simulink model "ALL_JP360_DBW_V6_5_1103"  (R2022a)
settings: Solver=FixedStepAuto  StartTime=0.0  StopTime=inf  FixedStep=0.01  RelTol=1e-3  EnableMultiTasking=on
model workspace (MAT data in the model file):
  g = 9.8
undefined symbols (not defined in the file or in its folder): canChannel, delta_v_p, IPM_Line_C0, IPM_Line_C1, IPM_Line_C2, IPM_Line_C3, M, M_p, MRR_ObjDistX, MRR_ObjDistY, MRR_ObjFusionCamID, MRR_ObjFusionSig, MRR_ObjID, MRR_ObjRelVelX, MRR_ObjRelVelY, MRR_ObjType, MRR_ObjUpdFlg, none, obj_vaild, untracktime, V, videoinput
libraries: canfdmsglib x230, canfdlib x76, slpidlib x24, simulink x18, dspstat3 x14, ctrlSharedLib x1, simulink_extras x1, imaqlib x1, realtime_pacer_lib x1, dspvision x1, visionsinks x1
(part 39 of 55)

== system ALL_JP360_DBW_V6_5_1103/MsgFromCAN/SRR_ADCU_MsgFromCAN/SRR_ADCU_RRR_OBJPos9_0x1BC ==
  SRR_ADCU_RRR_OBJPos9_0x1BCFromInData : Inport  OutDataTypeStr=Bus:CAN_FD_MESSAGE_BUS
  Bus Creator : BusCreator  Inputs=42  OutDataTypeStr=Bus:SRR_ADCU_RRR_OBJPos9_0x1BC  NonVirtualBus=on
  CAN FD Unpack : canfdmsglib/CAN FD Unpack  CANdbFile=V363 SRR Private CAN-V1.3.dbc  MsgList=(none)  MsgName=RRR_OBJPos9_0x1BC  ProtocolMode=CAN FD  MsgIDType=Standard (11-bit identifier)  MsgIdentifier=444  MsgLength=48  SignalInfo={'RRR_CRCCheck_0x1BC','376','16','BE','unsigned','Standard','0','1','0','0','65535';'RRR_OBJ17_Dx','79','13','BE','unsigned','Standard','0','0.0625','-256','-256','255.938';'RRR_OBJ17_Dy','60','11','BE','unsigned','Standard','0','0.125','-128','-128','127.875';'RRR_OBJ17_ExistProb','112','6','BE','unsigned','Standard','0','2','0','0','100';'RRR_OBJ17_HeadingAngle','55','10','BE','unsigned','Standard','0','0.01','-3.14','-3.14','3.14';'RRR_OBJ17_Height','26','9','BE','unsigned','Standard','0','0.01','0','0','5.11';'RRR_OBJ17_Length','33','9','BE','unsigned','Standard','0','0.05','0','0','25.5';'RRR_OBJ17_Measured','126','2','BE','unsigned','Standard','0','1','0','0','3';'RRR_OBJ17_Motion_Status','162','3','BE','unsigned','Standard','0','1','0','0','7';'RRR_OBJ17_ObstacleProb','120','6','BE','unsigned','Standard','0','2','0','0','100';'RRR_OBJ17_RefPointDx','144','13','BE','unsigned','Standard','0','0.0625','-256','-256','255.938';'RRR_OBJ17_RefPointDy','141','11','BE','unsigned','Standard','0','0.125','-128','-128','127.875';'RRR_OBJ17_RefPointLoc','157','3','BE','unsigned','Standard','0','1','0','0','7';'RRR_OBJ17_RelAx','118','9','BE','unsigned','Standard','0','0.0625','-16','-16','15.9375';'RRR_OBJ17_RelAy','111','10','BE','unsigned','Standard','0','0.03125','-16','-16','15.9688';'RRR_OBJ17_RelVx','89','12','BE','unsigned','Standard','0','0.0625','-128','-128','127.938';'RRR_OBJ17_RelVy','85','10','BE','unsigned','Standard','0','0.125','-64','-64','63.875';'RRR_OBJ17_Track_Age','165','8','BE','unsigned','Standard','0','1','0','0','255';'RRR_OBJ17_Track_ID','1','7','BE','unsigned','Standard','0','1','0','0','127';'RRR_OBJ17_Type','14','3','BE','unsigned','Standard','0','1','0','0','7';'RRR_OBJ17_Width','19','11','BE','unsigned','Standard','0','0.01','0','0','12';'RRR_OBJ18_Dx','247','13','BE','unsigned','Standard','0','0.0625','-256','-256','255.938';'RRR_OBJ18_Dy','228','11','BE','unsigned','Standard','0','0.125','-128','-128','127.875';'RRR_OBJ18_ExistProb','280','6','BE','unsigned','Standard','0','2','0','0','100';'RRR_OBJ18_HeadingAngle','223','10','BE','unsigned','Standard','0','0.01','-3.14','-3.14','3.14';'RRR_OBJ18_Height','194','9','BE','unsigned','Standard','0','0.01','0','0','5.11';'RRR_OBJ18_Length','201','9','BE','unsigned','Standard','0','0.05','0','0','25.5';'RRR_OBJ18_Measured','294','2','BE','unsigned','Standard','0','1','0','0','3';'RRR_OBJ18_Motion_Status','330','3','BE','unsigned','Standard','0','1','0','0','7';'RRR_OBJ18_ObstacleProb','288','6','BE','unsigned','Standard','0','2','0','0','100';'RRR_OBJ18_RefPointDx','312','13','BE','unsigned','Standard','0','0.0625','-256','-256','255.938';'RRR_OBJ18_RefPointDy','309','11','BE','unsigned','Standard','0','0.125','-128','-128','127.875';'RRR_OBJ18_RefPointLoc','325','3','BE','unsigned','Standard','0','1','0','0','7';'RRR_OBJ18_RelAx','286','9','BE','unsigned','Standard','0','0.0625','-16','-16','15.9375';'RRR_OBJ18_RelAy','279','10','BE','unsigned','Standard','0','0.03125','-16','-16','15.9688';'RRR_OBJ18_RelVx','257','12','BE','unsigned','Standard','0','0.0625','-128','-128','127.938';'RRR_OBJ18_RelVy','253','10','BE','unsigned','Standard','0','0.125','-64','-64','63.875';'RRR_OBJ18_Track_Age','333','8','BE','unsigned','Standard','0','1','0','0','255';'RRR_OBJ18_Track_ID','169','7','BE','unsigned','Standard','0','1','0','0','127';'RRR_OBJ18_Type','182','3','BE','unsigned','Standard','0','1','0','0','7';'RRR_OBJ18_Width','187','11','BE','unsigned','Standard','0','0.01','0','0','12';'RRR_RollingCounter_0x1BC','360','4','BE','unsigned','Standard','0','1','0','0','15'}  IDPort=off  TimestampPort=off  ErrorPort=off  RemotePort=off  LengthPort=off  StatusPort=off  BRSPort=off  ESIPort=off  DLCPort=off  ApplyMinMax=off
      settings: SourceProductBaseCode=ME,XP,VN  DataFormat=CANdb specified signals
  Data Type Conversion1 : DataTypeConversion  OutDataTypeStr=uint16  SaturateOnIntegerOverflow=off  RndMeth=Floor
  Data Type Conversion{4,8..10,13,19..20,24,28..30,33,39..40,42} (15 alike) : DataTypeConversion  OutDataTypeStr=int8  SaturateOnIntegerOverflow=off  RndMeth=Floor
  Data Type Conversion{2..3,5..7,11..12,14..17,21..23,25..27,31..32,34..37,41} (24 alike) : DataTypeConversion  OutDataTypeStr=single  SaturateOnIntegerOverflow=off  RndMeth=Floor
  Data Type Conversion18 : DataTypeConversion  OutDataTypeStr=uint8  SaturateOnIntegerOverflow=off  RndMeth=Floor
  Data Type Conversion38 : DataTypeConversion  OutDataTypeStr=uint8  SaturateOnIntegerOverflow=off  RndMeth=Floor
  SRR_ADCU_RRR_OBJPos9_0x1BCFromOutData : Outport  OutDataTypeStr=Bus:SRR_ADCU_RRR_OBJPos9_0x1BC
  wires:
  CAN FD Unpack/1 -> Data Type Conversion1/1
  CAN FD Unpack/2 -> Data Type Conversion2/1
  CAN FD Unpack/3 -> Data Type Conversion3/1
  CAN FD Unpack/4 -> Data Type Conversion4/1
  CAN FD Unpack/5 -> Data Type Conversion5/1
  CAN FD Unpack/6 -> Data Type Conversion6/1
  CAN FD Unpack/7 -> Data Type Conversion7/1
  CAN FD Unpack/8 -> Data Type Conversion8/1
  CAN FD Unpack/9 -> Data Type Conversion9/1
  CAN FD Unpack/10 -> Data Type Conversion10/1
  CAN FD Unpack/11 -> Data Type Conversion11/1
  CAN FD Unpack/12 -> Data Type Conversion12/1
  CAN FD Unpack/13 -> Data Type Conversion13/1
  CAN FD Unpack/14 -> Data Type Conversion14/1
  CAN FD Unpack/15 -> Data Type Conversion15/1
  CAN FD Unpack/16 -> Data Type Conversion16/1
  CAN FD Unpack/17 -> Data Type Conversion17/1
  CAN FD Unpack/18 -> Data Type Conversion18/1
  CAN FD Unpack/19 -> Data Type Conversion19/1
  CAN FD Unpack/20 -> Data Type Conversion20/1
  CAN FD Unpack/21 -> Data Type Conversion21/1
  CAN FD Unpack/22 -> Data Type Conversion22/1
  CAN FD Unpack/23 -> Data Type Conversion23/1
  CAN FD Unpack/24 -> Data Type Conversion24/1
  CAN FD Unpack/25 -> Data Type Conversion25/1
  CAN FD Unpack/26 -> Data Type Conversion26/1
  CAN FD Unpack/27 -> Data Type Conversion27/1
  CAN FD Unpack/28 -> Data Type Conversion28/1
  CAN FD Unpack/29 -> Data Type Conversion29/1
  CAN FD Unpack/30 -> Data Type Conversion30/1
  CAN FD Unpack/31 -> Data Type Conversion31/1
  CAN FD Unpack/32 -> Data Type Conversion32/1
  CAN FD Unpack/33 -> Data Type Conversion33/1
  CAN FD Unpack/34 -> Data Type Conversion34/1
  CAN FD Unpack/35 -> Data Type Conversion35/1
  CAN FD Unpack/36 -> Data Type Conversion36/1
  CAN FD Unpack/37 -> Data Type Conversion37/1
  CAN FD Unpack/38 -> Data Type Conversion38/1
  CAN FD Unpack/39 -> Data Type Conversion39/1
  CAN FD Unpack/40 -> Data Type Conversion40/1
  CAN FD Unpack/41 -> Data Type Conversion41/1
  CAN FD Unpack/42 -> Data Type Conversion42/1
  Data Type Conversion1/1 -> Bus Creator/1  "RRR_CRCCheck_0x1BC"
  Data Type Conversion2/1 -> Bus Creator/2  "RRR_OBJ17_Dx"
  Data Type Conversion3/1 -> Bus Creator/3  "RRR_OBJ17_Dy"
  Data Type Conversion4/1 -> Bus Creator/4  "RRR_OBJ17_ExistProb"
  Data Type Conversion5/1 -> Bus Creator/5  "RRR_OBJ17_HeadingAngle"
  Data Type Conversion6/1 -> Bus Creator/6  "RRR_OBJ17_Height"
  Data Type Conversion7/1 -> Bus Creator/7  "RRR_OBJ17_Length"
  Data Type Conversion8/1 -> Bus Creator/8  "RRR_OBJ17_Measured"
  Data Type Conversion9/1 -> Bus Creator/9  "RRR_OBJ17_Motion_Status"
  Data Type Conversion10/1 -> Bus Creator/10  "RRR_OBJ17_ObstacleProb"
  Data Type Conversion11/1 -> Bus Creator/11  "RRR_OBJ17_RefPointDx"
  Data Type Conversion12/1 -> Bus Creator/12  "RRR_OBJ17_RefPointDy"
  Data Type Conversion13/1 -> Bus Creator/13  "RRR_OBJ17_RefPointLoc"
  Data Type Conversion14/1 -> Bus Creator/14  "RRR_OBJ17_RelAx"
  Data Type Conversion15/1 -> Bus Creator/15  "RRR_OBJ17_RelAy"
  Data Type Conversion16/1 -> Bus Creator/16  "RRR_OBJ17_RelVx"
  Data Type Conversion17/1 -> Bus Creator/17  "RRR_OBJ17_RelVy"
  Data Type Conversion18/1 -> Bus Creator/18  "RRR_OBJ17_Track_Age"
  Data Type Conversion19/1 -> Bus Creator/19  "RRR_OBJ17_Track_ID"
  Data Type Conversion20/1 -> Bus Creator/20  "RRR_OBJ17_Type"
  Data Type Conversion21/1 -> Bus Creator/21  "RRR_OBJ17_Width"
  Data Type Conversion22/1 -> Bus Creator/22  "RRR_OBJ18_Dx"
  Data Type Conversion23/1 -> Bus Creator/23  "RRR_OBJ18_Dy"
  Data Type Conversion24/1 -> Bus Creator/24  "RRR_OBJ18_ExistProb"
  Data Type Conversion25/1 -> Bus Creator/25  "RRR_OBJ18_HeadingAngle"
  Data Type Conversion26/1 -> Bus Creator/26  "RRR_OBJ18_Height"
  Data Type Conversion27/1 -> Bus Creator/27  "RRR_OBJ18_Length"
  Data Type Conversion28/1 -> Bus Creator/28  "RRR_OBJ18_Measured"
  Data Type Conversion29/1 -> Bus Creator/29  "RRR_OBJ18_Motion_Status"
  Data Type Conversion30/1 -> Bus Creator/30  "RRR_OBJ18_ObstacleProb"
  Data Type Conversion31/1 -> Bus Creator/31  "RRR_OBJ18_RefPointDx"
  Data Type Conversion32/1 -> Bus Creator/32  "RRR_OBJ18_RefPointDy"
  Data Type Conversion33/1 -> Bus Creator/33  "RRR_OBJ18_RefPointLoc"
  Data Type Conversion34/1 -> Bus Creator/34  "RRR_OBJ18_RelAx"
  Data Type Conversion35/1 -> Bus Creator/35  "RRR_OBJ18_RelAy"
  Data Type Conversion36/1 -> Bus Creator/36  "RRR_OBJ18_RelVx"
  Data Type Conversion37/1 -> Bus Creator/37  "RRR_OBJ18_RelVy"
  Data Type Conversion38/1 -> Bus Creator/38  "RRR_OBJ18_Track_Age"
  Data Type Conversion39/1 -> Bus Creator/39  "RRR_OBJ18_Track_ID"
  Data Type Conversion40/1 -> Bus Creator/40  "RRR_OBJ18_Type"
  Data Type Conversion41/1 -> Bus Creator/41  "RRR_OBJ18_Width"
  Data Type Conversion42/1 -> Bus Creator/42  "RRR_RollingCounter_0x1BC"
  Bus Creator/1 -> SRR_ADCU_RRR_OBJPos9_0x1BCFromOutData/1  "SRR_ADCU_RRR_OBJPos9_0x1BCFromOutData"
  SRR_ADCU_RRR_OBJPos9_0x1BCFromInData/1 -> CAN FD Unpack/1  "SRR_ADCU_RRR_OBJPos9_0x1BCFromInData"

== system ALL_JP360_DBW_V6_5_1103/MsgFromCAN/Subsystem/Subsystem1 ==
  VR_ADCU_MRR_ObjHeader_0x680FromOutData : Inport
  Bus Selector : BusSelector  OutputSignals=MRR_ObjDistX_03,MRR_ObjDistY_03,MRR_ObjExistProb_03,MRR_ObjFusionCamID_03,MRR_ObjFusionSig_03,MRR_ObjID_03,MRR_ObjMovingSts_03,MRR_ObjObstacleProb_03,MRR_ObjRelAccelX_03,MRR_ObjRelAccelY_03,MRR_ObjRelVelX_03,MRR_ObjRelVelY_03,MRR_ObjType_03,MRR_ObjUpdFlg_03
  Bus Selector1 : BusSelector  OutputSignals=MRR_ObjDistX_04,MRR_ObjDistY_04,MRR_ObjExistProb_04,MRR_ObjFusionCamID_04,MRR_ObjFusionSig_04,MRR_ObjID_04,MRR_ObjMovingSts_04,MRR_ObjObstacleProb_04,MRR_ObjRelAccelX_04,MRR_ObjRelAccelY_04,MRR_ObjRelVelX_04,MRR_ObjRelVelY_04,MRR_ObjType_04,MRR_ObjUpdFlg_04
  Data Type Conversion{,1..27} (28 alike) : DataTypeConversion  OutDataTypeStr=single  SaturateOnIntegerOverflow=off  RndMeth=Floor
  Mux : Mux  Inputs=14
  Mux1 : Mux  Inputs=14
  Out1 : Outport
  Out2 : Outport  Port=2
  wires:
  Data Type Conversion26/1 -> Mux1/13
  Data Type Conversion24/1 -> Mux1/11
  Data Type Conversion22/1 -> Mux1/9
  Data Type Conversion20/1 -> Mux1/7
  Data Type Conversion27/1 -> Mux1/14
  Data Type Conversion25/1 -> Mux1/12
  Data Type Conversion23/1 -> Mux1/10
  Data Type Conversion21/1 -> Mux1/8
  Data Type Conversion13/1 -> Mux/14
  Data Type Conversion15/1 -> Mux1/2
  Data Type Conversion17/1 -> Mux1/4
  Data Type Conversion19/1 -> Mux1/6
  Data Type Conversion2/1 -> Mux/3
  Data Type Conversion14/1 -> Mux1/1
  Data Type Conversion16/1 -> Mux1/3
  Data Type Conversion18/1 -> Mux1/5
  Bus Selector1/10 -> Data Type Conversion23/1  "<MRR_ObjRelAccelY_04>"
  Bus Selector1/12 -> Data Type Conversion25/1  "<MRR_ObjRelVelY_04>"
  Bus Selector1/14 -> Data Type Conversion27/1  "<MRR_ObjUpdFlg_04>"
  Bus Selector1/11 -> Data Type Conversion24/1  "<MRR_ObjRelVelX_04>"
  Bus Selector1/13 -> Data Type Conversion26/1  "<MRR_ObjType_04>"
  Bus Selector1/5 -> Data Type Conversion18/1  "<MRR_ObjFusionSig_04>"
  Bus Selector1/7 -> Data Type Conversion20/1  "<MRR_ObjMovingSts_04>"
  Bus Selector1/9 -> Data Type Conversion22/1  "<MRR_ObjRelAccelX_04>"
  Bus Selector/14 -> Data Type Conversion13/1  "<MRR_ObjUpdFlg_03>"
  Bus Selector1/4 -> Data Type Conversion17/1  "<MRR_ObjFusionCamID_04>"
  Bus Selector1/6 -> Data Type Conversion19/1  "<MRR_ObjID_04>"
  Bus Selector1/8 -> Data Type Conversion21/1  "<MRR_ObjObstacleProb_04>"
  Bus Selector1/3 -> Data Type Conversion16/1  "<MRR_ObjExistProb_04>"
  Bus Selector/6 -> Data Type Conversion5/1  "<MRR_ObjID_03>"
  Bus Selector/8 -> Data Type Conversion7/1  "<MRR_ObjObstacleProb_03>"
  Bus Selector/10 -> Data Type Conversion9/1  "<MRR_ObjRelAccelY_03>"
  Bus Selector/12 -> Data Type Conversion11/1  "<MRR_ObjRelVelY_03>"
  Bus Selector1/2 -> Data Type Conversion15/1  "<MRR_ObjDistY_04>"
  VR_ADCU_MRR_ObjHeader_0x680FromOutData/1 -> Bus Selector/1, Bus Selector1/1
  Bus Selector/1 -> Data Type Conversion/1  "<MRR_ObjDistX_03>"
  Bus Selector1/1 -> Data Type Conversion14/1  "<MRR_ObjDistX_04>"
  Data Type Conversion/1 -> Mux/1
  Data Type Conversion10/1 -> Mux/11
  Data Type Conversion12/1 -> Mux/13
  Data Type Conversion1/1 -> Mux/2
  Data Type Conversion11/1 -> Mux/12
  Data Type Conversion3/1 -> Mux/4
  Data Type Conversion5/1 -> Mux/6
  Data Type Conversion7/1 -> Mux/8
  Data Type Conversion9/1 -> Mux/10
  Data Type Conversion4/1 -> Mux/5
  Data Type Conversion6/1 -> Mux/7
  Data Type Conversion8/1 -> Mux/9
  Bus Selector/7 -> Data Type Conversion6/1  "<MRR_ObjMovingSts_03>"
  Bus Selector/9 -> Data Type Conversion8/1  "<MRR_ObjRelAccelX_03>"
  Bus Selector/11 -> Data Type Conversion10/1  "<MRR_ObjRelVelX_03>"
  Bus Selector/13 -> Data Type Conversion12/1  "<MRR_ObjType_03>"
  Bus Selector/5 -> Data Type Conversion4/1  "<MRR_ObjFusionSig_03>"
  Bus Selector/4 -> Data Type Conversion3/1  "<MRR_ObjFusionCamID_03>"
  Bus Selector/3 -> Data Type Conversion2/1  "<MRR_ObjExistProb_03>"
  Bus Selector/2 -> Data Type Conversion1/1  "<MRR_ObjDistY_03>"
  Mux1/1 -> Out2/1
  Mux/1 -> Out1/1

== system ALL_JP360_DBW_V6_5_1103/MsgFromCAN/Subsystem/Subsystem10 ==
  VR_ADCU_MRR_ObjHeader_0x680FromOutData : Inport
  Bus Selector : BusSelector  OutputSignals=MRR_ObjDistX_21,MRR_ObjDistY_21,MRR_ObjExistProb_21,MRR_ObjFusionCamID_21,MRR_ObjFusionSig_21,MRR_ObjID_21,MRR_ObjMovingSts_21,MRR_ObjObstacleProb_21,MRR_ObjRelAccelX_21,MRR_ObjRelAccelY_21,MRR_ObjRelVelX_21,MRR_ObjRelVelY_21,MRR_ObjType_21,MRR_ObjUpdFlg_21
  Bus Selector1 : BusSelector  OutputSignals=MRR_ObjDistX_22,MRR_ObjDistY_22,MRR_ObjExistProb_22,MRR_ObjFusionCamID_22,MRR_ObjFusionSig_22,MRR_ObjID_22,MRR_ObjMovingSts_22,MRR_ObjObstacleProb_22,MRR_ObjRelAccelX_22,MRR_ObjRelAccelY_22,MRR_ObjRelVelX_22,MRR_ObjRelVelY_22,MRR_ObjType_22,MRR_ObjUpdFlg_22
  Data Type Conversion{,1..27} (28 alike) : DataTypeConversion  OutDataTypeStr=single  SaturateOnIntegerOverflow=off  RndMeth=Floor
  Mux : Mux  Inputs=14
  Mux1 : Mux  Inputs=14
  Out1 : Outport
  Out2 : Outport  Port=2
  wires:
  Data Type Conversion3/1 -> Mux/4
  Data Type Conversion26/1 -> Mux1/12
  Data Type Conversion24/1 -> Mux1/10
  Data Type Conversion22/1 -> Mux1/8
  Data Type Conversion4/1 -> Mux/5
  Data Type Conversion27/1 -> Mux1/13
  Data Type Conversion25/1 -> Mux1/11
  Data Type Conversion23/1 -> Mux1/9
  Data Type Conversion15/1 -> Mux1/1
  Data Type Conversion17/1 -> Mux1/3
  Data Type Conversion19/1 -> Mux1/5
  Data Type Conversion20/1 -> Mux1/6
  Data Type Conversion2/1 -> Mux/3
  Data Type Conversion16/1 -> Mux1/2
  Data Type Conversion18/1 -> Mux1/4
  Data Type Conversion21/1 -> Mux1/7
  Bus Selector1/13 -> Data Type Conversion27/1  "<MRR_ObjType_22>"
  Bus Selector1/12 -> Data Type Conversion26/1  "<MRR_ObjRelVelY_22>"
  Bus Selector1/5 -> Data Type Conversion19/1  "<MRR_ObjFusionSig_22>"
  Bus Selector1/7 -> Data Type Conversion21/1  "<MRR_ObjMovingSts_22>"
  Bus Selector1/9 -> Data Type Conversion23/1  "<MRR_ObjRelAccelX_22>"
  Bus Selector1/11 -> Data Type Conversion25/1  "<MRR_ObjRelVelX_22>"
  Bus Selector1/4 -> Data Type Conversion18/1  "<MRR_ObjFusionCamID_22>"
  Bus Selector1/6 -> Data Type Conversion20/1  "<MRR_ObjID_22>"
  Bus Selector1/8 -> Data Type Conversion22/1  "<MRR_ObjObstacleProb_22>"
  Bus Selector1/10 -> Data Type Conversion24/1  "<MRR_ObjRelAccelY_22>"
  Bus Selector/1 -> Data Type Conversion/1  "<MRR_ObjDistX_21>"
  Bus Selector1/3 -> Data Type Conversion17/1  "<MRR_ObjExistProb_22>"
  Bus Selector1/2 -> Data Type Conversion16/1  "<MRR_ObjDistY_22>"
  Data Type Conversion12/1 -> Mux/13
  Data Type Conversion10/1 -> Mux/11
  Data Type Conversion/1 -> Mux/1
  Bus Selector1/1 -> Data Type Conversion15/1  "<MRR_ObjDistX_22>"
  Bus Selector/2 -> Data Type Conversion1/1  "<MRR_ObjDistY_21>"
  Data Type Conversion13/1 -> Mux/14
  Data Type Conversion11/1 -> Mux/12
  Data Type Conversion1/1 -> Mux/2
  Data Type Conversion9/1 -> Mux/10
  Data Type Conversion7/1 -> Mux/8
  Data Type Conversion5/1 -> Mux/6
  Data Type Conversion8/1 -> Mux/9
  Data Type Conversion6/1 -> Mux/7
  Bus Selector/3 -> Data Type Conversion2/1  "<MRR_ObjExistProb_21>"
  Bus Selector/6 -> Data Type Conversion5/1  "<MRR_ObjID_21>"
  Bus Selector/4 -> Data Type Conversion3/1  "<MRR_ObjFusionCamID_21>"
  Bus Selector/7 -> Data Type Conversion6/1  "<MRR_ObjMovingSts_21>"
  Bus Selector/5 -> Data Type Conversion4/1  "<MRR_ObjFusionSig_21>"
  Bus Selector/14 -> Data Type Conversion13/1  "<MRR_ObjUpdFlg_21>"
  Bus Selector/12 -> Data Type Conversion11/1  "<MRR_ObjRelVelY_21>"
  Bus Selector/10 -> Data Type Conversion9/1  "<MRR_ObjRelAccelY_21>"
  Bus Selector/8 -> Data Type Conversion7/1  "<MRR_ObjObstacleProb_21>"
  Bus Selector/13 -> Data Type Conversion12/1  "<MRR_ObjType_21>"
  Bus Selector/11 -> Data Type Conversion10/1  "<MRR_ObjRelVelX_21>"
  Bus Selector/9 -> Data Type Conversion8/1  "<MRR_ObjRelAccelX_21>"
  Mux/1 -> Out1/1
  Mux1/1 -> Out2/1
  VR_ADCU_MRR_ObjHeader_0x680FromOutData/1 -> Bus Selector1/1, Bus Selector/1

== system ALL_JP360_DBW_V6_5_1103/MsgFromCAN/Subsystem/Subsystem11 ==
  VR_ADCU_MRR_ObjHeader_0x680FromOutData : Inport
  Bus Selector : BusSelector  OutputSignals=MRR_ObjDistX_23,MRR_ObjDistY_23,MRR_ObjExistProb_23,MRR_ObjFusionCamID_23,MRR_ObjFusionSig_23,MRR_ObjID_23,MRR_ObjMovingSts_23,MRR_ObjObstacleProb_23,MRR_ObjRelAccelX_23,MRR_ObjRelAccelY_23,MRR_ObjRelVelX_23,MRR_ObjRelVelY_23,MRR_ObjType_23,MRR_ObjUpdFlg_23
  Bus Selector1 : BusSelector  OutputSignals=MRR_ObjDistX_24,MRR_ObjDistY_24,MRR_ObjExistProb_24,MRR_ObjFusionCamID_24,MRR_ObjFusionSig_24,MRR_ObjID_24,MRR_ObjMovingSts_24,MRR_ObjObstacleProb_24,MRR_ObjRelAccelX_24,MRR_ObjRelAccelY_24,MRR_ObjRelVelX_24,MRR_ObjRelVelY_24,MRR_ObjType_24,MRR_ObjUpdFlg_24
  Data Type Conversion{,1..27} (28 alike) : DataTypeConversion  OutDataTypeStr=single  SaturateOnIntegerOverflow=off  RndMeth=Floor
  Mux : Mux  Inputs=14
  Mux1 : Mux  Inputs=14
  Out1 : Outport
  Out2 : Outport  Port=2
  wires:
  Bus Selector/3 -> Data Type Conversion2/1  "<MRR_ObjExistProb_23>"
  Data Type Conversion8/1 -> Mux/9
  Data Type Conversion6/1 -> Mux/7
  Data Type Conversion4/1 -> Mux/5
  Data Type Conversion27/1 -> Mux1/14
  Data Type Conversion26/1 -> Mux1/13
  Data Type Conversion24/1 -> Mux1/11
  Data Type Conversion22/1 -> Mux1/9
  Data Type Conversion20/1 -> Mux1/7
  Data Type Conversion2/1 -> Mux/3
  Data Type Conversion25/1 -> Mux1/12
  Data Type Conversion23/1 -> Mux1/10
  Data Type Conversion21/1 -> Mux1/8
  Data Type Conversion13/1 -> Mux/14
  Data Type Conversion15/1 -> Mux1/2
  Data Type Conversion17/1 -> Mux1/4
  Data Type Conversion19/1 -> Mux1/6
  Data Type Conversion12/1 -> Mux/13
  Data Type Conversion14/1 -> Mux1/1
  Data Type Conversion16/1 -> Mux1/3
  Data Type Conversion18/1 -> Mux1/5
  Bus Selector1/14 -> Data Type Conversion27/1  "<MRR_ObjUpdFlg_24>"
  Bus Selector1/2 -> Data Type Conversion15/1  "<MRR_ObjDistY_24>"
  Bus Selector1/7 -> Data Type Conversion20/1  "<MRR_ObjMovingSts_24>"
  Bus Selector1/9 -> Data Type Conversion22/1  "<MRR_ObjRelAccelX_24>"
  Bus Selector1/11 -> Data Type Conversion24/1  "<MRR_ObjRelVelX_24>"
  Bus Selector1/13 -> Data Type Conversion26/1  "<MRR_ObjType_24>"
  Bus Selector1/6 -> Data Type Conversion19/1  "<MRR_ObjID_24>"
  Bus Selector1/8 -> Data Type Conversion21/1  "<MRR_ObjObstacleProb_24>"
  Bus Selector1/10 -> Data Type Conversion23/1  "<MRR_ObjRelAccelY_24>"
  Bus Selector1/12 -> Data Type Conversion25/1  "<MRR_ObjRelVelY_24>"
  Bus Selector/13 -> Data Type Conversion12/1  "<MRR_ObjType_23>"
  Bus Selector/11 -> Data Type Conversion10/1  "<MRR_ObjRelVelX_23>"
  Bus Selector1/5 -> Data Type Conversion18/1  "<MRR_ObjFusionSig_24>"
  Bus Selector/14 -> Data Type Conversion13/1  "<MRR_ObjUpdFlg_23>"
  Bus Selector/12 -> Data Type Conversion11/1  "<MRR_ObjRelVelY_23>"
  Bus Selector/10 -> Data Type Conversion9/1  "<MRR_ObjRelAccelY_23>"
  Bus Selector1/4 -> Data Type Conversion17/1  "<MRR_ObjFusionCamID_24>"
  VR_ADCU_MRR_ObjHeader_0x680FromOutData/1 -> Bus Selector/1, Bus Selector1/1
  Bus Selector1/3 -> Data Type Conversion16/1  "<MRR_ObjExistProb_24>"
  Mux/1 -> Out1/1
  Bus Selector1/1 -> Data Type Conversion14/1  "<MRR_ObjDistX_24>"
  Data Type Conversion10/1 -> Mux/11
  Data Type Conversion/1 -> Mux/1
  Data Type Conversion11/1 -> Mux/12
  Data Type Conversion1/1 -> Mux/2
  Data Type Conversion9/1 -> Mux/10
  Data Type Conversion7/1 -> Mux/8
  Data Type Conversion5/1 -> Mux/6
  Data Type Conversion3/1 -> Mux/4
  Bus Selector/1 -> Data Type Conversion/1  "<MRR_ObjDistX_23>"
  Bus Selector/2 -> Data Type Conversion1/1  "<MRR_ObjDistY_23>"
  Bus Selector/8 -> Data Type Conversion7/1  "<MRR_ObjObstacleProb_23>"
  Bus Selector/6 -> Data Type Conversion5/1  "<MRR_ObjID_23>"
  Bus Selector/4 -> Data Type Conversion3/1  "<MRR_ObjFusionCamID_23>"
  Bus Selector/9 -> Data Type Conversion8/1  "<MRR_ObjRelAccelX_23>"
  Bus Selector/7 -> Data Type Conversion6/1  "<MRR_ObjMovingSts_23>"
  Bus Selector/5 -> Data Type Conversion4/1  "<MRR_ObjFusionSig_23>"
  Mux1/1 -> Out2/1

== system ALL_JP360_DBW_V6_5_1103/MsgFromCAN/Subsystem/Subsystem12 ==
  VR_ADCU_MRR_ObjHeader_0x680FromOutData : Inport
  Bus Selector : BusSelector  OutputSignals=MRR_ObjDistX_25,MRR_ObjDistY_25,MRR_ObjExistProb_25,MRR_ObjFusionCamID_25,MRR_ObjFusionSig_25,MRR_ObjID_25,MRR_ObjMovingSts_25,MRR_ObjObstacleProb_25,MRR_ObjRelAccelX_25,MRR_ObjRelAccelY_25,MRR_ObjRelVelX_25,MRR_ObjRelVelY_25,MRR_ObjType_25,MRR_ObjUpdFlg_25
  Bus Selector1 : BusSelector  OutputSignals=MRR_ObjDistX_26,MRR_ObjDistY_26,MRR_ObjExistProb_26,MRR_ObjFusionCamID_26,MRR_ObjFusionSig_26,MRR_ObjID_26,MRR_ObjMovingSts_26,MRR_ObjObstacleProb_26,MRR_ObjRelAccelX_26,MRR_ObjRelAccelY_26,MRR_ObjRelVelX_26,MRR_ObjRelVelY_26,MRR_ObjType_26,MRR_ObjUpdFlg_26
  Data Type Conversion{,1..27} (28 alike) : DataTypeConversion  OutDataTypeStr=single  SaturateOnIntegerOverflow=off  RndMeth=Floor
  Mux : Mux  Inputs=14
  Mux1 : Mux  Inputs=14
  Out1 : Outport
  Out2 : Outport  Port=2
  wires:
  Data Type Conversion27/1 -> Mux1/14
  Data Type Conversion25/1 -> Mux1/12
  Data Type Conversion23/1 -> Mux1/10
  Data Type Conversion21/1 -> Mux1/8
  VR_ADCU_MRR_ObjHeader_0x680FromOutData/1 -> Bus Selector1/1, Bus Selector/1
  Mux1/1 -> Out2/1
  Mux/1 -> Out1/1
  Data Type Conversion3/1 -> Mux/4
  Data Type Conversion26/1 -> Mux1/13
  Data Type Conversion24/1 -> Mux1/11
  Data Type Conversion22/1 -> Mux1/9
  Data Type Conversion15/1 -> Mux1/2
  Data Type Conversion17/1 -> Mux1/4
  Data Type Conversion19/1 -> Mux1/6
  Data Type Conversion20/1 -> Mux1/7
  Data Type Conversion2/1 -> Mux/3
  Data Type Conversion14/1 -> Mux1/1
  Data Type Conversion16/1 -> Mux1/3
  Data Type Conversion18/1 -> Mux1/5
  Bus Selector1/3 -> Data Type Conversion16/1  "<MRR_ObjExistProb_26>"
  Bus Selector1/8 -> Data Type Conversion21/1  "<MRR_ObjObstacleProb_26>"
  Bus Selector1/10 -> Data Type Conversion23/1  "<MRR_ObjRelAccelY_26>"
  Bus Selector1/12 -> Data Type Conversion25/1  "<MRR_ObjRelVelY_26>"
  Bus Selector1/14 -> Data Type Conversion27/1  "<MRR_ObjUpdFlg_26>"
  Bus Selector/1 -> Data Type Conversion/1  "<MRR_ObjDistX_25>"
  Bus Selector1/9 -> Data Type Conversion22/1  "<MRR_ObjRelAccelX_26>"
  Bus Selector1/11 -> Data Type Conversion24/1  "<MRR_ObjRelVelX_26>"
  Bus Selector1/13 -> Data Type Conversion26/1  "<MRR_ObjType_26>"
  Bus Selector/13 -> Data Type Conversion12/1  "<MRR_ObjType_25>"
  Bus Selector1/5 -> Data Type Conversion18/1  "<MRR_ObjFusionSig_26>"
  Bus Selector1/7 -> Data Type Conversion20/1  "<MRR_ObjMovingSts_26>"
  Bus Selector/14 -> Data Type Conversion13/1  "<MRR_ObjUpdFlg_25>"
  Bus Selector/12 -> Data Type Conversion11/1  "<MRR_ObjRelVelY_25>"
  Bus Selector1/4 -> Data Type Conversion17/1  "<MRR_ObjFusionCamID_26>"
  Bus Selector1/6 -> Data Type Conversion19/1  "<MRR_ObjID_26>"
  Bus Selector1/2 -> Data Type Conversion15/1  "<MRR_ObjDistY_26>"
  Bus Selector1/1 -> Data Type Conversion14/1  "<MRR_ObjDistX_26>"
  Data Type Conversion12/1 -> Mux/13
  Data Type Conversion10/1 -> Mux/11
  Data Type Conversion/1 -> Mux/1
  Data Type Conversion13/1 -> Mux/14
  Data Type Conversion11/1 -> Mux/12
  Data Type Conversion1/1 -> Mux/2
  Data Type Conversion8/1 -> Mux/9
  Data Type Conversion6/1 -> Mux/7
  Data Type Conversion4/1 -> Mux/5
  Data Type Conversion9/1 -> Mux/10
  Data Type Conversion7/1 -> Mux/8
  Data Type Conversion5/1 -> Mux/6
  Bus Selector/2 -> Data Type Conversion1/1  "<MRR_ObjDistY_25>"
  Bus Selector/3 -> Data Type Conversion2/1  "<MRR_ObjExistProb_25>"
  Bus Selector/10 -> Data Type Conversion9/1  "<MRR_ObjRelAccelY_25>"
  Bus Selector/8 -> Data Type Conversion7/1  "<MRR_ObjObstacleProb_25>"
  Bus Selector/6 -> Data Type Conversion5/1  "<MRR_ObjID_25>"
  Bus Selector/4 -> Data Type Conversion3/1  "<MRR_ObjFusionCamID_25>"
  Bus Selector/11 -> Data Type Conversion10/1  "<MRR_ObjRelVelX_25>"
  Bus Selector/9 -> Data Type Conversion8/1  "<MRR_ObjRelAccelX_25>"
  Bus Selector/7 -> Data Type Conversion6/1  "<MRR_ObjMovingSts_25>"
  Bus Selector/5 -> Data Type Conversion4/1  "<MRR_ObjFusionSig_25>"

== system ALL_JP360_DBW_V6_5_1103/MsgFromCAN/Subsystem/Subsystem13 ==
  VR_ADCU_MRR_ObjHeader_0x680FromOutData : Inport
  Bus Selector : BusSelector  OutputSignals=MRR_ObjDistX_27,MRR_ObjDistY_27,MRR_ObjExistProb_27,MRR_ObjFusionCamID_27,MRR_ObjFusionSig_27,MRR_ObjID_27,MRR_ObjMovingSts_27,MRR_ObjObstacleProb_27,MRR_ObjRelAccelX_27,MRR_ObjRelAccelY_27,MRR_ObjRelVelX_27,MRR_ObjRelVelY_27,MRR_ObjType_27,MRR_ObjUpdFlg_27
  Bus Selector1 : BusSelector  OutputSignals=MRR_ObjDistX_28,MRR_ObjDistY_28,MRR_ObjExistProb_28,MRR_ObjFusionCamID_28,MRR_ObjFusionSig_28,MRR_ObjID_28,MRR_ObjMovingSts_28,MRR_ObjObstacleProb_28,MRR_ObjRelAccelX_28,MRR_ObjRelAccelY_28,MRR_ObjRelVelX_28,MRR_ObjRelVelY_28,MRR_ObjType_28,MRR_ObjUpdFlg_28
  Data Type Conversion{,1..27} (28 alike) : DataTypeConversion  OutDataTypeStr=single  SaturateOnIntegerOverflow=off  RndMeth=Floor
  Mux : Mux  Inputs=14
  Mux1 : Mux  Inputs=14
  Out1 : Outport
  Out2 : Outport  Port=2
  wires:
  Data Type Conversion5/1 -> Mux/6
  Data Type Conversion3/1 -> Mux/4
  Data Type Conversion26/1 -> Mux1/13
  Data Type Conversion24/1 -> Mux1/11
  Data Type Conversion6/1 -> Mux/7
  Data Type Conversion4/1 -> Mux/5
  Data Type Conversion27/1 -> Mux1/14
  Data Type Conversion25/1 -> Mux1/12
  Data Type Conversion17/1 -> Mux1/4
  Data Type Conversion19/1 -> Mux1/6
  Data Type Conversion22/1 -> Mux1/9
  Data Type Conversion20/1 -> Mux1/7
  Data Type Conversion2/1 -> Mux/3
  Data Type Conversion18/1 -> Mux1/5
  Data Type Conversion23/1 -> Mux1/10
  Data Type Conversion21/1 -> Mux1/8
  VR_ADCU_MRR_ObjHeader_0x680FromOutData/1 -> Bus Selector/1, Bus Selector1/1
  Data Type Conversion12/1 -> Mux/13
  Data Type Conversion10/1 -> Mux/11
  Data Type Conversion14/1 -> Mux1/1
  Data Type Conversion16/1 -> Mux1/3
  Data Type Conversion13/1 -> Mux/14
  Data Type Conversion11/1 -> Mux/12
  Data Type Conversion1/1 -> Mux/2
  Data Type Conversion15/1 -> Mux1/2
  Bus Selector1/10 -> Data Type Conversion23/1  "<MRR_ObjRelAccelY_28>"
  Bus Selector1/12 -> Data Type Conversion25/1  "<MRR_ObjRelVelY_28>"
  Bus Selector1/14 -> Data Type Conversion27/1  "<MRR_ObjUpdFlg_28>"
  Bus Selector1/11 -> Data Type Conversion24/1  "<MRR_ObjRelVelX_28>"
  Bus Selector1/13 -> Data Type Conversion26/1  "<MRR_ObjType_28>"
  Bus Selector1/5 -> Data Type Conversion18/1  "<MRR_ObjFusionSig_28>"
  Bus Selector1/7 -> Data Type Conversion20/1  "<MRR_ObjMovingSts_28>"
  Bus Selector1/9 -> Data Type Conversion22/1  "<MRR_ObjRelAccelX_28>"
  Bus Selector/14 -> Data Type Conversion13/1  "<MRR_ObjUpdFlg_27>"
  Bus Selector/1 -> Data Type Conversion/1  "<MRR_ObjDistX_27>"
  Bus Selector1/4 -> Data Type Conversion17/1  "<MRR_ObjFusionCamID_28>"
  Bus Selector1/6 -> Data Type Conversion19/1  "<MRR_ObjID_28>"
  Bus Selector1/8 -> Data Type Conversion21/1  "<MRR_ObjObstacleProb_28>"
  Data Type Conversion/1 -> Mux/1
  Bus Selector1/3 -> Data Type Conversion16/1  "<MRR_ObjExistProb_28>"
  Bus Selector1/2 -> Data Type Conversion15/1  "<MRR_ObjDistY_28>"
  Bus Selector1/1 -> Data Type Conversion14/1  "<MRR_ObjDistX_28>"
  Data Type Conversion9/1 -> Mux/10
  Data Type Conversion7/1 -> Mux/8
  Data Type Conversion8/1 -> Mux/9
  Bus Selector/12 -> Data Type Conversion11/1  "<MRR_ObjRelVelY_27>"
  Bus Selector/10 -> Data Type Conversion9/1  "<MRR_ObjRelAccelY_27>"
  Bus Selector/8 -> Data Type Conversion7/1  "<MRR_ObjObstacleProb_27>"
  Bus Selector/6 -> Data Type Conversion5/1  "<MRR_ObjID_27>"
  Bus Selector/2 -> Data Type Conversion1/1  "<MRR_ObjDistY_27>"
  Bus Selector/3 -> Data Type Conversion2/1  "<MRR_ObjExistProb_27>"
  Mux/1 -> Out1/1
  Bus Selector/4 -> Data Type Conversion3/1  "<MRR_ObjFusionCamID_27>"
  Bus Selector/5 -> Data Type Conversion4/1  "<MRR_ObjFusionSig_27>"
  Bus Selector/13 -> Data Type Conversion12/1  "<MRR_ObjType_27>"
  Bus Selector/11 -> Data Type Conversion10/1  "<MRR_ObjRelVelX_27>"
  Bus Selector/9 -> Data Type Conversion8/1  "<MRR_ObjRelAccelX_27>"
  Bus Selector/7 -> Data Type Conversion6/1  "<MRR_ObjMovingSts_27>"
  Mux1/1 -> Out2/1

== system ALL_JP360_DBW_V6_5_1103/MsgFromCAN/Subsystem/Subsystem14 ==
  VR_ADCU_MRR_ObjHeader_0x680FromOutData : Inport
  Bus Selector : BusSelector  OutputSignals=MRR_ObjDistX_29,MRR_ObjDistY_29,MRR_ObjExistProb_29,MRR_ObjFusionCamID_29,MRR_ObjFusionSig_29,MRR_ObjID_29,MRR_ObjMovingSts_29,MRR_ObjObstacleProb_29,MRR_ObjRelAccelX_29,MRR_ObjRelAccelY_29,MRR_ObjRelVelX_29,MRR_ObjRelVelY_29,MRR_ObjType_29,MRR_ObjUpdFlg_29
  Bus Selector1 : BusSelector  OutputSignals=MRR_ObjDistX_30,MRR_ObjDistY_30,MRR_ObjExistProb_30,MRR_ObjFusionCamID_30,MRR_ObjFusionSig_30,MRR_ObjID_30,MRR_ObjMovingSts_30,MRR_ObjObstacleProb_30,MRR_ObjRelAccelX_30,MRR_ObjRelAccelY_30,MRR_ObjRelVelX_30,MRR_ObjRelVelY_30,MRR_ObjType_30,MRR_ObjUpdFlg_30
  Data Type Conversion{,1..27} (28 alike) : DataTypeConversion  OutDataTypeStr=single  SaturateOnIntegerOverflow=off  RndMeth=Floor
  Mux : Mux  Inputs=14
  Mux1 : Mux  Inputs=14
  Out1 : Outport
  Out2 : Outport  Port=2
  wires:
  Mux/1 -> Out1/1
  Mux1/1 -> Out2/1
  VR_ADCU_MRR_ObjHeader_0x680FromOutData/1 -> Bus Selector/1, Bus Selector1/1
  Bus Selector/9 -> Data Type Conversion8/1  "<MRR_ObjRelAccelX_29>"
  Bus Selector/10 -> Data Type Conversion9/1  "<MRR_ObjRelAccelY_29>"
  Bus Selector/8 -> Data Type Conversion7/1  "<MRR_ObjObstacleProb_29>"
  Bus Selector/11 -> Data Type Conversion10/1  "<MRR_ObjRelVelX_29>"
  Bus Selector/7 -> Data Type Conversion6/1  "<MRR_ObjMovingSts_29>"
  Bus Selector/12 -> Data Type Conversion11/1  "<MRR_ObjRelVelY_29>"
  Bus Selector/6 -> Data Type Conversion5/1  "<MRR_ObjID_29>"
  Bus Selector/13 -> Data Type Conversion12/1  "<MRR_ObjType_29>"
  Bus Selector/5 -> Data Type Conversion4/1  "<MRR_ObjFusionSig_29>"
  Bus Selector/14 -> Data Type Conversion13/1  "<MRR_ObjUpdFlg_29>"
  Bus Selector/4 -> Data Type Conversion3/1  "<MRR_ObjFusionCamID_29>"
  Bus Selector/3 -> Data Type Conversion2/1  "<MRR_ObjExistProb_29>"
  Bus Selector/2 -> Data Type Conversion1/1  "<MRR_ObjDistY_29>"
  Bus Selector/1 -> Data Type Conversion/1  "<MRR_ObjDistX_29>"
  Data Type Conversion8/1 -> Mux/9
  Data Type Conversion9/1 -> Mux/10
  Data Type Conversion7/1 -> Mux/8
  Data Type Conversion10/1 -> Mux/11
  Data Type Conversion6/1 -> Mux/7
  Data Type Conversion11/1 -> Mux/12
  Data Type Conversion5/1 -> Mux/6
  Data Type Conversion12/1 -> Mux/13
  Data Type Conversion4/1 -> Mux/5
  Data Type Conversion13/1 -> Mux/14
  Data Type Conversion3/1 -> Mux/4
  Data Type Conversion2/1 -> Mux/3
  Data Type Conversion1/1 -> Mux/2
  Data Type Conversion/1 -> Mux/1
  Bus Selector1/1 -> Data Type Conversion14/1  "<MRR_ObjDistX_30>"
  Bus Selector1/2 -> Data Type Conversion15/1  "<MRR_ObjDistY_30>"
  Bus Selector1/3 -> Data Type Conversion16/1  "<MRR_ObjExistProb_30>"
  Bus Selector1/4 -> Data Type Conversion17/1  "<MRR_ObjFusionCamID_30>"
  Bus Selector1/5 -> Data Type Conversion18/1  "<MRR_ObjFusionSig_30>"
  Bus Selector1/6 -> Data Type Conversion19/1  "<MRR_ObjID_30>"
  Bus Selector1/7 -> Data Type Conversion20/1  "<MRR_ObjMovingSts_30>"
  Bus Selector1/8 -> Data Type Conversion21/1  "<MRR_ObjObstacleProb_30>"
  Bus Selector1/9 -> Data Type Conversion22/1  "<MRR_ObjRelAccelX_30>"
  Bus Selector1/10 -> Data Type Conversion23/1  "<MRR_ObjRelAccelY_30>"
  Bus Selector1/11 -> Data Type Conversion24/1  "<MRR_ObjRelVelX_30>"
  Bus Selector1/12 -> Data Type Conversion25/1  "<MRR_ObjRelVelY_30>"
  Bus Selector1/13 -> Data Type Conversion26/1  "<MRR_ObjType_30>"
  Bus Selector1/14 -> Data Type Conversion27/1  "<MRR_ObjUpdFlg_30>"
  Data Type Conversion14/1 -> Mux1/1
  Data Type Conversion15/1 -> Mux1/2
  Data Type Conversion16/1 -> Mux1/3
  Data Type Conversion17/1 -> Mux1/4
  Data Type Conversion18/1 -> Mux1/5
  Data Type Conversion19/1 -> Mux1/6
  Data Type Conversion20/1 -> Mux1/7
  Data Type Conversion21/1 -> Mux1/8
  Data Type Conversion22/1 -> Mux1/9
  Data Type Conversion23/1 -> Mux1/10
  Data Type Conversion24/1 -> Mux1/11
  Data Type Conversion25/1 -> Mux1/12
  Data Type Conversion26/1 -> Mux1/13
  Data Type Conversion27/1 -> Mux1/14

== system ALL_JP360_DBW_V6_5_1103/MsgFromCAN/Subsystem/Subsystem15 ==
  VR_ADCU_MRR_ObjHeader_0x680FromOutData : Inport
  Bus Selector : BusSelector  OutputSignals=MRR_ObjDistX_31,MRR_ObjDistY_31,MRR_ObjExistProb_31,MRR_ObjFusionCamID_31,MRR_ObjFusionSig_31,MRR_ObjID_31,MRR_ObjMovingSts_31,MRR_ObjObstacleProb_31,MRR_ObjRelAccelX_31,MRR_ObjRelAccelY_31,MRR_ObjRelVelX_31,MRR_ObjRelVelY_31,MRR_ObjType_31,MRR_ObjUpdFlg_31
  Bus Selector1 : BusSelector  OutputSignals=MRR_ObjDistX_32,MRR_ObjDistY_32,MRR_ObjExistProb_32,MRR_ObjFusionCamID_32,MRR_ObjFusionSig_32,MRR_ObjID_32,MRR_ObjMovingSts_32,MRR_ObjObstacleProb_32,MRR_ObjRelAccelX_32,MRR_ObjRelAccelY_32,MRR_ObjRelVelX_32,MRR_ObjRelVelY_32,MRR_ObjType_32,MRR_ObjUpdFlg_32
  Data Type Conversion{,1..27} (28 alike) : DataTypeConversion  OutDataTypeStr=single  SaturateOnIntegerOverflow=off  RndMeth=Floor
  Mux : Mux  Inputs=14
  Mux1 : Mux  Inputs=14
  Out1 : Outport
  Out2 : Outport  Port=2
  wires:
  VR_ADCU_MRR_ObjHeader_0x680FromOutData/1 -> Bus Selector/1, Bus Selector1/1
  Mux1/1 -> Out2/1
  Mux/1 -> Out1/1
  Bus Selector/9 -> Data Type Conversion8/1  "<MRR_ObjRelAccelX_31>"
  Bus Selector/8 -> Data Type Conversion7/1  "<MRR_ObjObstacleProb_31>"
  Bus Selector/10 -> Data Type Conversion9/1  "<MRR_ObjRelAccelY_31>"
  Bus Selector/7 -> Data Type Conversion6/1  "<MRR_ObjMovingSts_31>"
  Bus Selector/11 -> Data Type Conversion10/1  "<MRR_ObjRelVelX_31>"
  Bus Selector/6 -> Data Type Conversion5/1  "<MRR_ObjID_31>"
  Bus Selector/12 -> Data Type Conversion11/1  "<MRR_ObjRelVelY_31>"
  Bus Selector/5 -> Data Type Conversion4/1  "<MRR_ObjFusionSig_31>"
  Bus Selector/13 -> Data Type Conversion12/1  "<MRR_ObjType_31>"
  Bus Selector/4 -> Data Type Conversion3/1  "<MRR_ObjFusionCamID_31>"
  Bus Selector/14 -> Data Type Conversion13/1  "<MRR_ObjUpdFlg_31>"
  Bus Selector/3 -> Data Type Conversion2/1  "<MRR_ObjExistProb_31>"
  Bus Selector/2 -> Data Type Conversion1/1  "<MRR_ObjDistY_31>"
  Bus Selector/1 -> Data Type Conversion/1  "<MRR_ObjDistX_31>"
  Data Type Conversion8/1 -> Mux/9
  Data Type Conversion7/1 -> Mux/8
  Data Type Conversion9/1 -> Mux/10
  Data Type Conversion6/1 -> Mux/7
  Data Type Conversion10/1 -> Mux/11
  Data Type Conversion5/1 -> Mux/6
  Data Type Conversion11/1 -> Mux/12
  Data Type Conversion4/1 -> Mux/5
  Data Type Conversion12/1 -> Mux/13
  Data Type Conversion3/1 -> Mux/4
  Data Type Conversion13/1 -> Mux/14
  Data Type Conversion2/1 -> Mux/3
  Data Type Conversion1/1 -> Mux/2
  Data Type Conversion/1 -> Mux/1
  Bus Selector1/1 -> Data Type Conversion14/1  "<MRR_ObjDistX_32>"
  Bus Selector1/2 -> Data Type Conversion15/1  "<MRR_ObjDistY_32>"
  Bus Selector1/3 -> Data Type Conversion16/1  "<MRR_ObjExistProb_32>"
  Bus Selector1/4 -> Data Type Conversion17/1  "<MRR_ObjFusionCamID_32>"
  Bus Selector1/5 -> Data Type Conversion18/1  "<MRR_ObjFusionSig_32>"
  Bus Selector1/6 -> Data Type Conversion19/1  "<MRR_ObjID_32>"
  Bus Selector1/7 -> Data Type Conversion20/1  "<MRR_ObjMovingSts_32>"
  Bus Selector1/8 -> Data Type Conversion21/1  "<MRR_ObjObstacleProb_32>"
  Bus Selector1/9 -> Data Type Conversion22/1  "<MRR_ObjRelAccelX_32>"
  Bus Selector1/10 -> Data Type Conversion23/1  "<MRR_ObjRelAccelY_32>"
  Bus Selector1/11 -> Data Type Conversion24/1  "<MRR_ObjRelVelX_32>"
  Bus Selector1/12 -> Data Type Conversion25/1  "<MRR_ObjRelVelY_32>"
  Bus Selector1/13 -> Data Type Conversion26/1  "<MRR_ObjType_32>"
  Bus Selector1/14 -> Data Type Conversion27/1  "<MRR_ObjUpdFlg_32>"
  Data Type Conversion14/1 -> Mux1/1
  Data Type Conversion15/1 -> Mux1/2
  Data Type Conversion16/1 -> Mux1/3
  Data Type Conversion17/1 -> Mux1/4
  Data Type Conversion18/1 -> Mux1/5
  Data Type Conversion19/1 -> Mux1/6
  Data Type Conversion20/1 -> Mux1/7
  Data Type Conversion21/1 -> Mux1/8
  Data Type Conversion22/1 -> Mux1/9
  Data Type Conversion23/1 -> Mux1/10
  Data Type Conversion24/1 -> Mux1/11
  Data Type Conversion25/1 -> Mux1/12
  Data Type Conversion26/1 -> Mux1/13
  Data Type Conversion27/1 -> Mux1/14

== system ALL_JP360_DBW_V6_5_1103/MsgFromCAN/Subsystem/Subsystem16 ==
  VR_ADCU_MRR_ObjHeader_0x680FromOutData : Inport
  Bus Selector : BusSelector  OutputSignals=MRR_ObjDistX_01,MRR_ObjDistY_01,MRR_ObjExistProb_01,MRR_ObjFusionCamID_01,MRR_ObjFusionSig_01,MRR_ObjID_01,MRR_ObjMovingSts_01,MRR_ObjObstacleProb_01,MRR_ObjRelAccelX_01,MRR_ObjRelAccelY_01,MRR_ObjRelVelX_01,MRR_ObjRelVelY_01,MRR_ObjType_01,MRR_ObjUpdFlg_01
  Bus Selector1 : BusSelector  OutputSignals=MRR_ObjDistX_02,MRR_ObjDistY_02,MRR_ObjExistProb_02,MRR_ObjFusionCamID_02,MRR_ObjFusionSig_02,MRR_ObjID_02,MRR_ObjMovingSts_02,MRR_ObjObstacleProb_02,MRR_ObjRelAccelX_02,MRR_ObjRelAccelY_02,MRR_ObjRelVelX_02,MRR_ObjRelVelY_02,MRR_ObjType_02,MRR_ObjUpdFlg_02
  Data Type Conversion{,1..27} (28 alike) : DataTypeConversion  OutDataTypeStr=single  SaturateOnIntegerOverflow=off  RndMeth=Floor
  Mux : Mux  Inputs=14
  Mux1 : Mux  Inputs=14
  Out1 : Outport
  Out2 : Outport  Port=2
  wires:
  Data Type Conversion14/1 -> Mux1/1
  Data Type Conversion18/1 -> Mux1/5
  Data Type Conversion17/1 -> Mux1/4
  Data Type Conversion16/1 -> Mux1/3
  Bus Selector/3 -> Data Type Conversion2/1  "<MRR_ObjExistProb_01>"
  Data Type Conversion15/1 -> Mux1/2
  Data Type Conversion21/1 -> Mux1/8
  Data Type Conversion20/1 -> Mux1/7
  Data Type Conversion23/1 -> Mux1/10
  Data Type Conversion19/1 -> Mux1/6
  Data Type Conversion22/1 -> Mux1/9
  Data Type Conversion24/1 -> Mux1/11
  Bus Selector/2 -> Data Type Conversion1/1  "<MRR_ObjDistY_01>"
  Data Type Conversion25/1 -> Mux1/12
  Data Type Conversion26/1 -> Mux1/13
  Data Type Conversion27/1 -> Mux1/14
  Bus Selector1/8 -> Data Type Conversion21/1  "<MRR_ObjObstacleProb_02>"
  Bus Selector1/10 -> Data Type Conversion23/1  "<MRR_ObjRelAccelY_02>"
  Bus Selector1/12 -> Data Type Conversion25/1  "<MRR_ObjRelVelY_02>"
  Bus Selector1/14 -> Data Type Conversion27/1  "<MRR_ObjUpdFlg_02>"
  Bus Selector1/9 -> Data Type Conversion22/1  "<MRR_ObjRelAccelX_02>"
  Bus Selector1/11 -> Data Type Conversion24/1  "<MRR_ObjRelVelX_02>"
  Bus Selector1/13 -> Data Type Conversion26/1  "<MRR_ObjType_02>"
  Bus Selector/13 -> Data Type Conversion12/1  "<MRR_ObjType_01>"
  Bus Selector1/5 -> Data Type Conversion18/1  "<MRR_ObjFusionSig_02>"
  Bus Selector1/7 -> Data Type Conversion20/1  "<MRR_ObjMovingSts_02>"
  Bus Selector/12 -> Data Type Conversion11/1  "<MRR_ObjRelVelY_01>"
  Bus Selector/14 -> Data Type Conversion13/1  "<MRR_ObjUpdFlg_01>"
  Bus Selector1/4 -> Data Type Conversion17/1  "<MRR_ObjFusionCamID_02>"
  Bus Selector1/6 -> Data Type Conversion19/1  "<MRR_ObjID_02>"
  Bus Selector1/3 -> Data Type Conversion16/1  "<MRR_ObjExistProb_02>"
  Bus Selector/1 -> Data Type Conversion/1  "<MRR_ObjDistX_01>"
  Bus Selector1/2 -> Data Type Conversion15/1  "<MRR_ObjDistY_02>"
  Bus Selector1/1 -> Data Type Conversion14/1  "<MRR_ObjDistX_02>"
  Data Type Conversion/1 -> Mux/1
  Data Type Conversion1/1 -> Mux/2
  Data Type Conversion6/1 -> Mux/7
  Data Type Conversion2/1 -> Mux/3
  Data Type Conversion3/1 -> Mux/4
  Data Type Conversion4/1 -> Mux/5
  Data Type Conversion5/1 -> Mux/6
  Data Type Conversion11/1 -> Mux/12
  Data Type Conversion7/1 -> Mux/8
  Data Type Conversion8/1 -> Mux/9
  Data Type Conversion9/1 -> Mux/10
  Data Type Conversion10/1 -> Mux/11
  Data Type Conversion12/1 -> Mux/13
  Data Type Conversion13/1 -> Mux/14
  Bus Selector/5 -> Data Type Conversion4/1  "<MRR_ObjFusionSig_01>"
  Bus Selector/7 -> Data Type Conversion6/1  "<MRR_ObjMovingSts_01>"
  Bus Selector/9 -> Data Type Conversion8/1  "<MRR_ObjRelAccelX_01>"
  Bus Selector/11 -> Data Type Conversion10/1  "<MRR_ObjRelVelX_01>"
  Bus Selector/4 -> Data Type Conversion3/1  "<MRR_ObjFusionCamID_01>"
  Bus Selector/6 -> Data Type Conversion5/1  "<MRR_ObjID_01>"
  Bus Selector/8 -> Data Type Conversion7/1  "<MRR_ObjObstacleProb_01>"
  Bus Selector/10 -> Data Type Conversion9/1  "<MRR_ObjRelAccelY_01>"
  Mux/1 -> Out1/1
  Mux1/1 -> Out2/1
  VR_ADCU_MRR_ObjHeader_0x680FromOutData/1 -> Bus Selector1/1, Bus Selector/1

== system ALL_JP360_DBW_V6_5_1103/MsgFromCAN/Subsystem/Subsystem2 ==
  VR_ADCU_MRR_ObjHeader_0x680FromOutData : Inport
  Bus Selector : BusSelector  OutputSignals=MRR_ObjDistX_05,MRR_ObjDistY_05,MRR_ObjExistProb_05,MRR_ObjFusionCamID_05,MRR_ObjFusionSig_05,MRR_ObjID_05,MRR_ObjMovingSts_05,MRR_ObjObstacleProb_05,MRR_ObjRelAccelX_05,MRR_ObjRelAccelY_05,MRR_ObjRelVelX_05,MRR_ObjRelVelY_05,MRR_ObjType_05,MRR_ObjUpdFlg_05
  Bus Selector1 : BusSelector  OutputSignals=MRR_ObjDistX_06,MRR_ObjDistY_06,MRR_ObjExistProb_06,MRR_ObjFusionCamID_06,MRR_ObjFusionSig_06,MRR_ObjID_06,MRR_ObjMovingSts_06,MRR_ObjObstacleProb_06,MRR_ObjRelAccelX_06,MRR_ObjRelAccelY_06,MRR_ObjRelVelX_06,MRR_ObjRelVelY_06,MRR_ObjType_06,MRR_ObjUpdFlg_06
  Data Type Conversion{,1..27} (28 alike) : DataTypeConversion  OutDataTypeStr=single  SaturateOnIntegerOverflow=off  RndMeth=Floor
  Mux : Mux  Inputs=14
  Mux1 : Mux  Inputs=14
  Mux2 : Mux  Inputs=14
  Out1 : Outport
  Out2 : Outport  Port=2
  wires:
  Bus Selector1/14 -> Data Type Conversion27/1  "<MRR_ObjUpdFlg_06>"
  Bus Selector1/12 -> Data Type Conversion25/1  "<MRR_ObjRelVelY_06>"
  Bus Selector1/10 -> Data Type Conversion23/1  "<MRR_ObjRelAccelY_06>"
  Bus Selector1/8 -> Data Type Conversion21/1  "<MRR_ObjObstacleProb_06>"
  Bus Selector1/13 -> Data Type Conversion26/1  "<MRR_ObjType_06>"
  Bus Selector1/11 -> Data Type Conversion24/1  "<MRR_ObjRelVelX_06>"
  Bus Selector1/9 -> Data Type Conversion22/1  "<MRR_ObjRelAccelX_06>"
  Bus Selector/13 -> Data Type Conversion12/1  "<MRR_ObjType_05>"
  Bus Selector1/5 -> Data Type Conversion18/1  "<MRR_ObjFusionSig_06>"
  Bus Selector1/7 -> Data Type Conversion20/1  "<MRR_ObjMovingSts_06>"
  Bus Selector/12 -> Data Type Conversion11/1  "<MRR_ObjRelVelY_05>"
  Bus Selector/14 -> Data Type Conversion13/1  "<MRR_ObjUpdFlg_05>"
  Bus Selector1/4 -> Data Type Conversion17/1  "<MRR_ObjFusionCamID_06>"
  Bus Selector1/6 -> Data Type Conversion19/1  "<MRR_ObjID_06>"
  Bus Selector/1 -> Data Type Conversion/1  "<MRR_ObjDistX_05>"
  Bus Selector1/3 -> Data Type Conversion16/1  "<MRR_ObjExistProb_06>"
  Bus Selector1/2 -> Data Type Conversion15/1  "<MRR_ObjDistY_06>"
  Bus Selector1/1 -> Data Type Conversion14/1  "<MRR_ObjDistX_06>"
  Data Type Conversion4/1 -> Mux/5
  Data Type Conversion23/1 -> Mux1/10
  Data Type Conversion25/1 -> Mux1/12
  Data Type Conversion27/1 -> Mux1/14
  Data Type Conversion3/1 -> Mux/4
  Data Type Conversion22/1 -> Mux1/9
  Data Type Conversion24/1 -> Mux1/11
  Data Type Conversion26/1 -> Mux1/13
  Data Type Conversion2/1 -> Mux/3
  Data Type Conversion16/1 -> Mux1/3
  Data Type Conversion18/1 -> Mux1/5
  Data Type Conversion21/1 -> Mux1/8
  Data Type Conversion15/1 -> Mux1/2
  Data Type Conversion17/1 -> Mux1/4
  Data Type Conversion19/1 -> Mux1/6
  Data Type Conversion20/1 -> Mux1/7
  Data Type Conversion12/1 -> Mux/13
  Data Type Conversion10/1 -> Mux/11
  Data Type Conversion/1 -> Mux/1
  Data Type Conversion14/1 -> Mux1/1
  Data Type Conversion11/1 -> Mux/12
  Data Type Conversion13/1 -> Mux/14
  Data Type Conversion1/1 -> Mux/2
  Data Type Conversion9/1 -> Mux/10
  Data Type Conversion7/1 -> Mux/8
  Data Type Conversion5/1 -> Mux/6
  Data Type Conversion8/1 -> Mux/9
  Data Type Conversion6/1 -> Mux/7
  Bus Selector/2 -> Data Type Conversion1/1  "<MRR_ObjDistY_05>"
  Bus Selector/3 -> Data Type Conversion2/1  "<MRR_ObjExistProb_05>"
  Bus Selector/10 -> Data Type Conversion9/1  "<MRR_ObjRelAccelY_05>"
  Bus Selector/8 -> Data Type Conversion7/1  "<MRR_ObjObstacleProb_05>"
  Bus Selector/6 -> Data Type Conversion5/1  "<MRR_ObjID_05>"
  Bus Selector/4 -> Data Type Conversion3/1  "<MRR_ObjFusionCamID_05>"
  Bus Selector/11 -> Data Type Conversion10/1  "<MRR_ObjRelVelX_05>"
  Bus Selector/9 -> Data Type Conversion8/1  "<MRR_ObjRelAccelX_05>"
  Bus Selector/7 -> Data Type Conversion6/1  "<MRR_ObjMovingSts_05>"
  Bus Selector/5 -> Data Type Conversion4/1  "<MRR_ObjFusionSig_05>"
  Mux1/1 -> Out2/1
  Mux/1 -> Out1/1
  VR_ADCU_MRR_ObjHeader_0x680FromOutData/1 -> Bus Selector/1, Bus Selector1/1
